simulink model "PID_controller"  (R2023a)
settings: Solver=VariableStepAuto  StartTime=0.0  StopTime=200  RelTol=1e-3
values from neighbouring files (symbols this model uses):
  dem = [taux 1]    [servo_simulation.m]
libraries: slpidlib x2
settings Model: Creator=PC  LastModifiedBy=PC

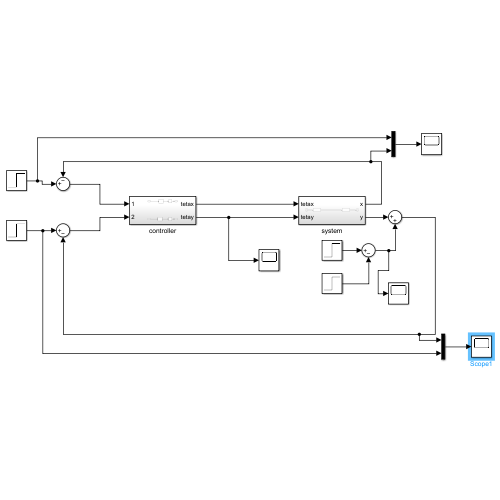
[thumbnail: Simulink's stored preview of the top-level diagram]
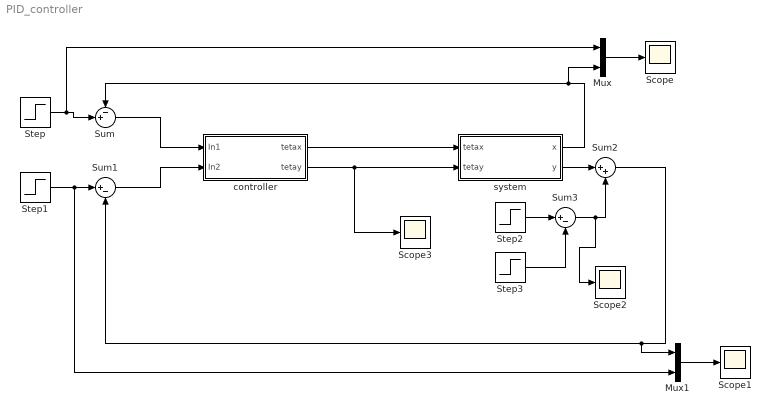
== system PID_controller ==
  Mux : Mux  Inputs=2
  Mux1 : Mux  Inputs=2
  Scope{,1..3} (4 alike) : Scope
  Step : Step  After=0  SampleTime=0
  Step1 : Step  After=30  SampleTime=0
  Step2 : Step  Time=40  After=4  SampleTime=0
  Step3 : Step  Time=45  After=4  SampleTime=0
  Sum : Sum  Inputs=-+|
  Sum1 : Sum  Inputs=|+-
  Sum2 : Sum  Inputs=|++
  Sum3 : Sum  Inputs=|+-
  controller : Subsystem
  system : Subsystem
  wires:
  Sum2/1 -> Sum1/2, Mux1/1
  system/1(x) -> Mux/2, Sum/1
  Sum3/1 -> Scope2/1, Sum2/2
  Step1/1 -> Mux1/2, Sum1/1
  system/2(y) -> Sum2/1
  controller/2(tetay) -> Scope3/1, system/2(tetay)
  Step/1 -> Mux/1, Sum/2
  Sum/1 -> controller/1(In1)
  Mux/1 -> Scope/1
  Mux1/1 -> Scope1/1
  Step3/1 -> Sum3/2
  Step2/1 -> Sum3/1
  controller/1(tetax) -> system/1(tetax)
  Sum1/1 -> controller/2(In2)

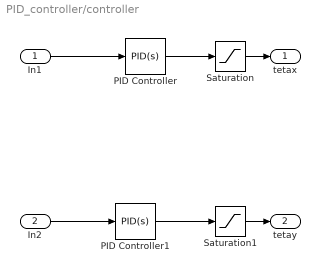
== system PID_controller/controller ==
  In1 : Inport
  In2 : Inport  Port=2
  PID Controller : slpidlib/PID Controller  Controller=PID  Form=Ideal  TimeDomain=Continuous-time  UseExternalTs=off  SampleTime=-1  IntegratorMethod=Forward Euler  FilterMethod=Forward Euler  ControllerParametersSource=internal  P=0.1656  I=1.1542  UseKiTs=off  D=2.2914  N=100  UseFilter=on  TunerSelectOption=Transfer Function Based (PID Tuner App)  InitialConditionSource=internal  InitialConditionForIntegrator=0  InitialConditionForFilter=0  DifferentiatorICPrevScaledInput=0  ExternalReset=none  TrackingMode=off  Kt=1  LimitOutput=off  SatLimitsSource=internal  UpperSaturationLimit=inf  LowerSaturationLimit=-inf  LinearizeAsGain=on  AntiWindupMode=none  Kb=1  LimitIntegrator=off  UpperIntegratorSaturationLimit=inf  LowerIntegratorSaturationLimit=-inf  POutMin=[]  POutMax=[]  IOutMin=[]  IOutMax=[]  DOutMin=[]  DOutMax=[]  NOutMin=[]  NOutMax=[]  SumOutMin=[]  SumOutMax=[]  SaturationOutMin=[]  SaturationOutMax=[]  PParamMin=[]  PParamMax=[]  IParamMin=[]  IParamMax=[]  DParamMin=[]  DParamMax=[]  NParamMin=[]  NParamMax=[]  KbParamMin=[]  KbParamMax=[]  KtParamMin=[]  KtParamMax=[]  KbOutMin=[]  KbOutMax=[]  KtOutMin=[]  KtOutMax=[]  IntegratorOutMin=[]  IntegratorOutMax=[]  FilterOutMin=[]  FilterOutMax=[]  SumI1OutMin=[]  SumI1OutMax=[]  SumI2OutMin=[]  SumI2OutMax=[]  SumI3OutMin=[]  SumI3OutMax=[]  SumI4OutMin=[]  SumI4OutMax=[]  SumDOutMin=[]  SumDOutMax=[]  DifferentiatorOutMin=[]  DifferentiatorOutMax=[]  FilterDiffOutCoefMin=[]  FilterDiffOutCoefMax=[]  ReciprocalOutMin=[]  ReciprocalOutMax=[]  SumDenOutMin=[]  SumDenOutMax=[]  SumNumOutMin=[]  SumNumOutMax=[]  DivideOutMin=[]  DivideOutMax=[]  UdiffTsProdOutMin=[]  UdiffTsProdOutMax=[]  NTsProdOutMin=[]  NTsProdOutMax=[]  UintegralTsProdOutMin=[]  UintegralTsProdOutMax=[]  UngainTsProdOutMin=[]  UngainTsProdOutMax=[]  ClampingZeroOutDataTypeStr=Inherit: Inherit via back propagation  ClampingZeroOutMin=[]  ClampingZeroOutMax=[]  FilterDenConstantOutDataTypeStr=Inherit: Inherit via back propagation  FilterDenConstantOutMin=[]  FilterDenConstantOutMax=[]  PCopyOutDataTypeStr=Inherit: Inherit via back propagation  PCopyOutMin=[]  PCopyOutMax=[]  NCopyOutDataTypeStr=Inherit: Inherit via back propagation  NCopyOutMin=[]  NCopyOutMax=[]  IntegratorContinuousStateAttributes=''  IntegratorStateMustResolveToSignalObject=off  IntegratorRTWStateStorageClass=Auto  FilterContinuousStateAttributes=''  FilterStateMustResolveToSignalObject=off  FilterRTWStateStorageClass=Auto  ParallelPVariant=Passthrough  IdealPVariant=InternalParameters  IVariant=InternalParameters  DVariant=InternalParameters  IntegratorVariant=Continuous  SatVariant=Disabled  AWVariant=Passthrough  PCopyVariant=Disabled  TRVariant=Disabled  FdbkBlocksVariant=Forward  IdealPFdbkVariant=Disabled  SatFdbkVariant=Disabled  DerivativeFilterVariant=ContFilter  NVariant=InternalParameters  NCopyVariant=Disabled  FilterICVariant=InternalICsFilter  IntegratorICVariant=InternalICs  ExternalResetVariant=Disabled  TRSumVariant=Passthrough  SumFdbkVariant=Disabled  SumVariant=Sum_PID  TsampFilterVariant=InternalTs  TsampNgainVariant=Passthrough  TsampIntegralVariant=Disabled_SignalSpec  ExternalSaturationOutDataTypeStr=Inherit: Same as second input
  PID Controller1 : slpidlib/PID Controller  Controller=PID  Form=Ideal  TimeDomain=Continuous-time  UseExternalTs=off  SampleTime=-1  IntegratorMethod=Forward Euler  FilterMethod=Forward Euler  ControllerParametersSource=internal  P=1  I=0.1  UseKiTs=off  D=1.5  N=100  UseFilter=on  TunerSelectOption=Frequency Response Based  InitialConditionSource=internal  InitialConditionForIntegrator=0  InitialConditionForFilter=0  DifferentiatorICPrevScaledInput=0  ExternalReset=none  TrackingMode=off  Kt=1  LimitOutput=off  SatLimitsSource=internal  UpperSaturationLimit=inf  LowerSaturationLimit=-inf  LinearizeAsGain=on  AntiWindupMode=none  Kb=1  LimitIntegrator=off  UpperIntegratorSaturationLimit=inf  LowerIntegratorSaturationLimit=-inf  POutMin=[]  POutMax=[]  IOutMin=[]  IOutMax=[]  DOutMin=[]  DOutMax=[]  NOutMin=[]  NOutMax=[]  SumOutMin=[]  SumOutMax=[]  SaturationOutMin=[]  SaturationOutMax=[]  PParamMin=[]  PParamMax=[]  IParamMin=[]  IParamMax=[]  DParamMin=[]  DParamMax=[]  NParamMin=[]  NParamMax=[]  KbParamMin=[]  KbParamMax=[]  KtParamMin=[]  KtParamMax=[]  KbOutMin=[]  KbOutMax=[]  KtOutMin=[]  KtOutMax=[]  IntegratorOutMin=[]  IntegratorOutMax=[]  FilterOutMin=[]  FilterOutMax=[]  SumI1OutMin=[]  SumI1OutMax=[]  SumI2OutMin=[]  SumI2OutMax=[]  SumI3OutMin=[]  SumI3OutMax=[]  SumI4OutMin=[]  SumI4OutMax=[]  SumDOutMin=[]  SumDOutMax=[]  DifferentiatorOutMin=[]  DifferentiatorOutMax=[]  FilterDiffOutCoefMin=[]  FilterDiffOutCoefMax=[]  ReciprocalOutMin=[]  ReciprocalOutMax=[]  SumDenOutMin=[]  SumDenOutMax=[]  SumNumOutMin=[]  SumNumOutMax=[]  DivideOutMin=[]  DivideOutMax=[]  UdiffTsProdOutMin=[]  UdiffTsProdOutMax=[]  NTsProdOutMin=[]  NTsProdOutMax=[]  UintegralTsProdOutMin=[]  UintegralTsProdOutMax=[]  UngainTsProdOutMin=[]  UngainTsProdOutMax=[]  ClampingZeroOutDataTypeStr=Inherit: Inherit via back propagation  ClampingZeroOutMin=[]  ClampingZeroOutMax=[]  FilterDenConstantOutDataTypeStr=Inherit: Inherit via back propagation  FilterDenConstantOutMin=[]  FilterDenConstantOutMax=[]  PCopyOutDataTypeStr=Inherit: Inherit via back propagation  PCopyOutMin=[]  PCopyOutMax=[]  NCopyOutDataTypeStr=Inherit: Inherit via back propagation  NCopyOutMin=[]  NCopyOutMax=[]  IntegratorContinuousStateAttributes=''  IntegratorStateMustResolveToSignalObject=off  IntegratorRTWStateStorageClass=Auto  FilterContinuousStateAttributes=''  FilterStateMustResolveToSignalObject=off  FilterRTWStateStorageClass=Auto  ParallelPVariant=Passthrough  IdealPVariant=InternalParameters  IVariant=InternalParameters  DVariant=InternalParameters  IntegratorVariant=Continuous  SatVariant=Disabled  AWVariant=Passthrough  PCopyVariant=Disabled  TRVariant=Disabled  FdbkBlocksVariant=Forward  IdealPFdbkVariant=Disabled  SatFdbkVariant=Disabled  DerivativeFilterVariant=ContFilter  NVariant=InternalParameters  NCopyVariant=Disabled  FilterICVariant=InternalICsFilter  IntegratorICVariant=InternalICs  ExternalResetVariant=Disabled  TRSumVariant=Passthrough  SumFdbkVariant=Disabled  SumVariant=Sum_PID  TsampFilterVariant=InternalTs  TsampNgainVariant=Passthrough  TsampIntegralVariant=Disabled_SignalSpec  ExternalSaturationOutDataTypeStr=Inherit: Same as second input
  Saturation : Saturate  UpperLimit=45  LowerLimit=-45
  Saturation1 : Saturate  UpperLimit=45  LowerLimit=-45
  tetax : Outport
  tetay : Outport  Port=2
  wires:
  In1/1 -> PID Controller/1
  Saturation/1 -> tetax/1
  PID Controller/1 -> Saturation/1
  Saturation1/1 -> tetay/1
  In2/1 -> PID Controller1/1
  PID Controller1/1 -> Saturation1/1

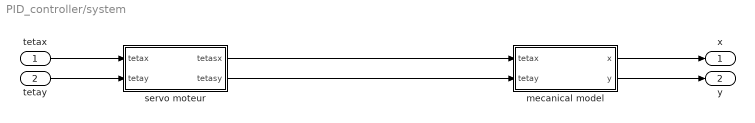
== system PID_controller/system ==
  tetax : Inport
  tetay : Inport  Port=2
  mecanical model : Subsystem
  servo moteur : Subsystem
  x : Outport
  y : Outport  Port=2
  wires:
  servo moteur/2(tetasy) -> mecanical model/2(tetay)
  servo moteur/1(tetasx) -> mecanical model/1(tetax)
  mecanical model/2(y) -> y/1
  mecanical model/1(x) -> x/1
  tetax/1 -> servo moteur/1(tetax)
  tetay/1 -> servo moteur/2(tetay)

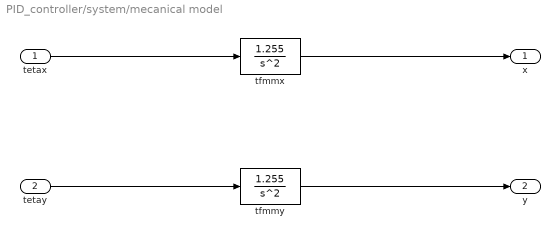
== system PID_controller/system/mecanical model ==
  tetax : Inport
  tetay : Inport  Port=2
  tfmmx : TransferFcn  Numerator=1.255  Denominator=[1 0 0]
  tfmmy : TransferFcn  Numerator=1.255  Denominator=[1 0 0]
  x : Outport
  y : Outport  Port=2
  wires:
  tetax/1 -> tfmmx/1
  tfmmx/1 -> x/1
  tetay/1 -> tfmmy/1
  tfmmy/1 -> y/1

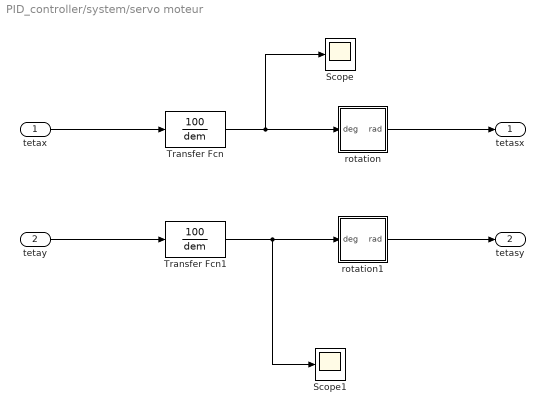
== system PID_controller/system/servo moteur ==
  tetax : Inport
  tetay : Inport  Port=2
  Scope : Scope
  Scope1 : Scope
  Transfer Fcn : TransferFcn  Numerator=100  Denominator=dem
  Transfer Fcn1 : TransferFcn  Numerator=100  Denominator=dem
  rotation : Subsystem
  rotation1 : Subsystem
  tetasx : Outport
  tetasy : Outport  Port=2
  wires:
  tetax/1 -> Transfer Fcn/1
  tetay/1 -> Transfer Fcn1/1
  Transfer Fcn/1 -> Scope/1, rotation/1(deg)
  rotation/1(rad) -> tetasx/1
  Transfer Fcn1/1 -> Scope1/1, rotation1/1(deg)
  rotation1/1(rad) -> tetasy/1

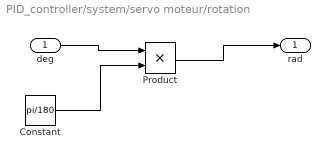
== system PID_controller/system/servo moteur/rotation ==
  deg : Inport
  Constant : Constant  Value=pi/180
  Product : Product
  rad : Outport
  wires:
  deg/1 -> Product/1
  Product/1 -> rad/1
  Constant/1 -> Product/2

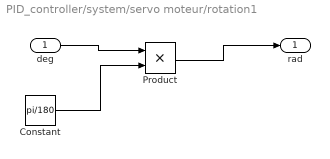
== system PID_controller/system/servo moteur/rotation1 ==
  deg : Inport
  Constant : Constant  Value=pi/180
  Product : Product
  rad : Outport
  wires:
  deg/1 -> Product/1
  Product/1 -> rad/1
  Constant/1 -> Product/2
